simulink model "cps_fmu_smoke_test"  (R2026a)
settings: Solver=FixedStepDiscrete  StopTime=0.01  FixedStep=1e-4
settings Model: Creator=CHUANCHAO  LastModifiedBy=CHUANCHAO

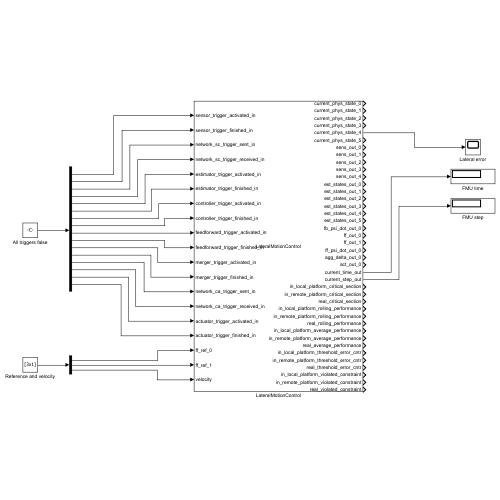
[thumbnail: Simulink's stored preview of the top-level diagram]
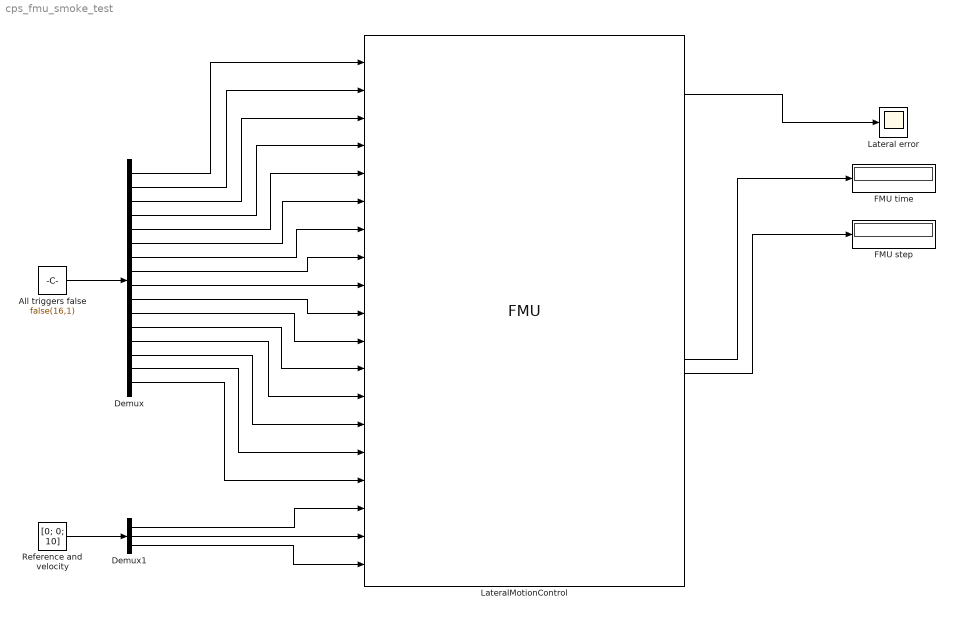
== system cps_fmu_smoke_test ==
  All triggers false : Constant  Value=false(16,1)  OutDataTypeStr=boolean  SampleTime=-1
  Demux : Demux  Outputs=16
  Demux1 : Demux  Outputs=3
  FMU step : Display
  FMU time : Display
  Lateral error : Scope
  LateralMotionControl : FMU  FMUName=LateralMotionControl.fmu  FMUMode=CoSimulation  FMUSampleTime=1e-4  FMUInitializeEnumObject=off  FMUCachedDialogLayout="{\"Geometry\":[1764,-1984,893,665],\"ParameterColumnsWidthConfig\":\"{\\\"columns\\\":[{\\\"name\\\":\\\"Parameter\\\",\\\"width\\\":148},{\\\"name\\\":\\\"Value\\\",\\\"width\\\":119},{\\\"name\\\":\\\"Unit\\\",\\\"width\\\":111},{\\\"name\\\":\\\"Description\\\",\\\"width\\\":327}]}\",\"InputColumnsWidthConfig\":\"{\\\"columns\\\":[{\\\"name\\\":\\\"Name\\\",\\\"width\\\":230},{\\\"name\\\":\\\"Visibility\\\",\\\"width\\\":60},{\\\"name\\\":\\\"Start\\\",\\\"width\\\":40},{\\\"name\\\":\\\"Unit\\\",\\\"width\\\":124},{\\\"name\\\":\\\"Type Object\\\",\\\"width\\\":169}]}\",\"OutputColumnsWidthConfig\":\"{\\\"columns\\\":[{\\\"name\\\":\\\"Name\\\",\\\"width\\\":48},{\\\"name\\\":\\\"Visibility\\\",\\\"width\\\":60},{\\\"name\\\":\\\"Start\\\",\\\"width\\\":40},{\\\"name\\\":\\\"Unit\\\",\\\"width\\\":36},{\\\"name\\\":\\\"Type Object\\\",\\\"width\\\":82}]}\"}"  K_trc_fb_0_0=-0.987  K_trc_fb_0_1=0.0  K_trc_fb_0_2=0.0  K_trc_fb_0_3=0.0  K_trc_fb_0_4=8.00  K_trc_fb_0_5=1.75  K_trc_ff_0_0=1.987  K_trc_ff_0_1=0.1974  K_yrc_x_0_0=-0.2876  K_yrc_x_0_1=0.0  K_yrc_x_0_2=1.0  K_yrc_x_0_3=0.0  K_yrc_x_0_4=0.0  K_yrc_x_0_5=0.0  K_yrc_psi_0_0=0.2876  x0_0=0.0  x0_1=0.0  x0_2=0.0  x0_3=0.0  x0_4=0.1  x0_5=0.0  noise_mean_0=0.0  noise_mean_1=0.0  noise_mean_2=0.0  noise_mean_3=0.0  noise_mean_4=0.0  noise_mean_5=0.0  noise_std_dev_0=0.0  noise_std_dev_1=0.0  noise_std_dev_2=0.0  noise_std_dev_3=0.0  noise_std_dev_4=0.0  noise_std_dev_5=0.0  init_velocity=10.0  mask(LateralMotionControl [Co-Simulation, v2.0]){}
      mask Display:
      | disp('LateralMotionControl');
      | port_label('output',1,'current_phys_state_0');
      | port_label('output',2,'current_phys_state_1');
      | port_label('output',3,'current_phys_state_2');
      | port_label('output',4,'current_phys_state_3');
      | port_label('output',5,'current_phys_state_4');
      | port_label('output',6,'current_phys_state_5');
      | port_label('output',7,'sens_out_0');
      | port_label('output',8,'sens_out_1');
      | port_label('output',9,'sens_out_2');
      | port_label('output',10,'sens_out_3');
      | port_label('output',11,'sens_out_4');
      | port_label('output',12,'est_states_out_0');
      | port_label('output',13,'est_states_out_1');
      | port_label('output',14,'est_states_out_2');
      | port_label('output',15,'est_states_out_3');
      | port_label('output',16,'est_states_out_4');
      | port_label('output',17,'est_states_out_5');
      | port_label('output',18,'fb_psi_dot_out_0');
      | port_label('output',19,'ff_out_0');
      | port_label('output',20,'ff_out_1');
      | port_label('output',21,'ff_psi_dot_out_0');
      | port_label('output',22,'agg_delta_out_0');
      | port_label('output',23,'act_out_0');
      | port_label('output',24,'current_time_out');
      | port_label('output',25,'current_step_out');
      | port_label('output',26,'in_local_platform_critical_section');
      | port_label('output',27,'in_remote_platform_critical_section');
      | port_label('output',28,'real_critical_section');
      | port_label('output',29,'in_local_platform_rolling_performance');
      | port_label('output',30,'in_remote_platform_rolling_performance');
      | port_label('output',31,'real_rolling_performance');
      | port_label('output',32,'in_local_platform_average_performance');
      | port_label('output',33,'in_remote_platform_average_performance');
      | port_label('output',34,'real_average_performance');
      | port_label('output',35,'in_local_platform_threshold_error_cntr');
      | port_label('output',36,'in_remote_platform_threshold_error_cntr');
      | port_label('output',37,'real_threshold_error_cntr');
      | port_label('output',38,'in_local_platform_violated_constraint');
      | port_label('output',39,'in_remote_platform_violated_constraint');
      | port_label('output',40,'real_violated_constraint');
      | port_label('input',1,'sensor_trigger_activated_in');
      | port_label('input',2,'sensor_trigger_finished_in');
      | port_label('input',3,'network_sc_trigger_sent_in');
      | port_label('input',4,'network_sc_trigger_received_in');
      | port_label('input',5,'estimator_trigger_activated_in');
      | port_label('input',6,'estimator_trigger_finished_in');
      | port_label('input',7,'controller_trigger_activated_in');
      | port_label('input',8,'controller_trigger_finished_in');
      | port_label('input',9,'feedforward_trigger_activated_in');
      | port_label('input',10,'feedforward_trigger_finished_in');
      | port_label('input',11,'merger_trigger_activated_in');
      | port_label('input',12,'merger_trigger_finished_in');
      | port_label('input',13,'network_ca_trigger_sent_in');
      | port_label('input',14,'network_ca_trigger_received_in');
      | port_label('input',15,'actuator_trigger_activated_in');
      | port_label('input',16,'actuator_trigger_finished_in');
      | port_label('input',17,'ff_ref_0');
      | port_label('input',18,'ff_ref_1');
      | port_label('input',19,'velocity');
  Reference and velocity : Constant  Value=[0; 0; 10]  OutDataTypeStr=double  SampleTime=-1
  wires:
  All triggers false/1 -> Demux/1
  Demux/1 -> LateralMotionControl/1
  Demux/2 -> LateralMotionControl/2
  Demux/3 -> LateralMotionControl/3
  Demux/4 -> LateralMotionControl/4
  Demux/5 -> LateralMotionControl/5
  Demux/6 -> LateralMotionControl/6
  Demux/7 -> LateralMotionControl/7
  Demux/8 -> LateralMotionControl/8
  Demux/9 -> LateralMotionControl/9
  Demux/10 -> LateralMotionControl/10
  Demux/11 -> LateralMotionControl/11
  Demux/12 -> LateralMotionControl/12
  Demux/13 -> LateralMotionControl/13
  Demux/14 -> LateralMotionControl/14
  Demux/15 -> LateralMotionControl/15
  Demux/16 -> LateralMotionControl/16
  Reference and velocity/1 -> Demux1/1
  Demux1/1 -> LateralMotionControl/17
  Demux1/2 -> LateralMotionControl/18
  Demux1/3 -> LateralMotionControl/19
  LateralMotionControl/24 -> FMU time/1
  LateralMotionControl/25 -> FMU step/1
  LateralMotionControl/5 -> Lateral error/1
